simulink model "forGenerate"  (R2015b)
settings: Solver=FixedStepAuto  StartTime=0  StopTime=13  FixedStep=10*(1e-3)  RelTol=1e-3
undefined symbols (not defined in the file or in its folder): qc
libraries: simulink x4
settings Model: Creator=acsl  LastModifiedBy=acsl
settings OptimizationCC: DefaultParameterBehavior=Inlined  UseFloatMulNetSlope=on  InlineInvariantSignals=on  PassReuseOutputArgsAs=Individual arguments  ZeroExternalMemoryAtStartup=off  ZeroInternalMemoryAtStartup=off  NoFixptDivByZeroProtection=on  EfficientFloat2IntCast=on  OptimizeModelRefInitCode=on  LifeSpan=1
settings HardwareCC: ProdBitPerPointer=32  ProdLargestAtomicInteger=Long  ProdLargestAtomicFloat=Double  ProdWordSize=32  ProdHWDeviceType=ARM Compatible->ARM Cortex
settings RTWCC: SystemTargetFile=ert.tlc  TemplateMakefile=ert_default_tmf  Description=Embedded Coder  GenerateReport=on  IncludeHyperlinkInReport=on  LaunchReport=on  GenerateTraceInfo=on  GenerateTraceReport=on  GenerateTraceReportSl=on  GenerateTraceReportSf=on  GenerateTraceReportEml=on  GenerateCodeMetricsReport=on
settings CodeAppCC: ForceParamTrailComments=on  IgnoreCustomStorageClasses=off  SimulinkDataObjDesc=on  CustomSymbolStrGlobalVar=rt$N$M  CustomSymbolStrType=$N$M  CustomSymbolStrFcn=$N$M$F  CustomSymbolStrMacro=$N$M  InsertBlockDesc=on
settings ERTTargetCC: GenerateSampleERTMain=on  IncludeMdlTerminateFcn=off  CombineSignalStateStructs=on  SupportContinuousTime=on  InlinedParameterPlacement=NonHierarchical  ERTCustomFileTemplate=example_file_process.tlc  ERTFilePackagingFormat=CompactWithDataFile

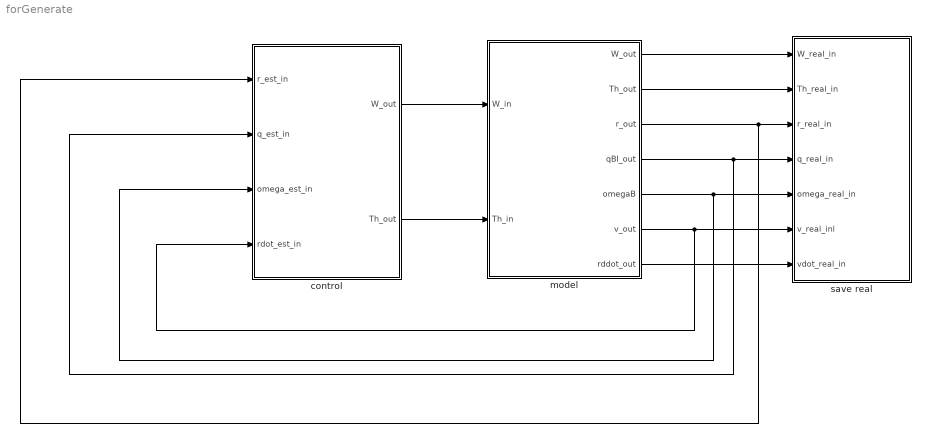
== system forGenerate ==
  control : Subsystem  InitFcn=init
  model : Subsystem
  save real : Subsystem
  wires:
  model/1(W_out) -> save real/1(W_real_in)
  model/2(Th_out) -> save real/2(Th_real_in)
  model/7(rddot_out) -> save real/7(vdot_real_in)
  model/5(omegaB) -> control/3(omega_est_in), save real/5(omega_real_in)
  control/1(W_out) -> model/1(W_in)
  control/2(Th_out) -> model/2(Th_in)
  model/3(r_out) -> control/1(r_est_in), save real/3(r_real_in)
  model/4(qBI_out) -> control/2(q_est_in), save real/4(q_real_in)
  model/6(v_out) -> control/4(rdot_est_in), save real/6(v_real_inl)

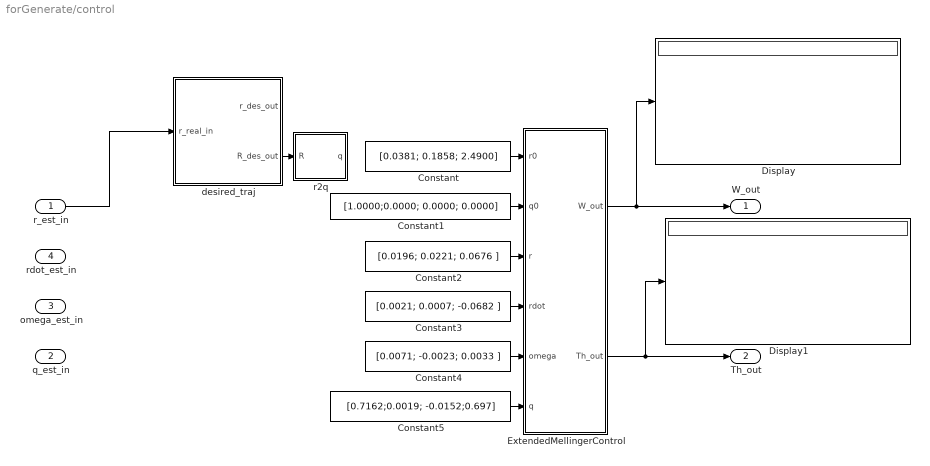
== system forGenerate/control ==
  r_est_in : Inport
  q_est_in : Inport  Port=2
  omega_est_in : Inport  Port=3
  rdot_est_in : Inport  Port=4
  Constant : Constant  Value=[0.0381; 0.1858; 2.4900]  VectorParams1D=off
  Constant1 : Constant  Value=[1.0000;0.0000; 0.0000; 0.0000]  VectorParams1D=off
  Constant2 : Constant  Value=[0.0196; 0.0221; 0.0676 ]  VectorParams1D=off
  Constant3 : Constant  Value=[0.0021; 0.0007; -0.0682 ]  VectorParams1D=off
  Constant4 : Constant  Value=[0.0071; -0.0023; 0.0033 ]
  Constant5 : Constant  Value=[0.7162;0.0019; -0.0152;0.697]  VectorParams1D=off
  Display : Display
  Display1 : Display
  ExtendedMellingerControl : Subsystem
  desired_traj : Subsystem
  r2q : MATLAB Function  TreatAsAtomicUnit=on
  W_out : Outport
  Th_out : Outport  Port=2
  wires:
  r_est_in/1 -> desired_traj/1(r_real_in)
  desired_traj/2(R_des_out) -> r2q/1(R)
  ExtendedMellingerControl/2(Th_out) -> Display1/1, Th_out/1
  Constant/1 -> ExtendedMellingerControl/1(r0)
  Constant1/1 -> ExtendedMellingerControl/2(q0)
  Constant2/1 -> ExtendedMellingerControl/3(r)
  Constant3/1 -> ExtendedMellingerControl/4(rdot)
  Constant4/1 -> ExtendedMellingerControl/5(omega)
  Constant5/1 -> ExtendedMellingerControl/6(q)
  ExtendedMellingerControl/1(W_out) -> Display/1, W_out/1

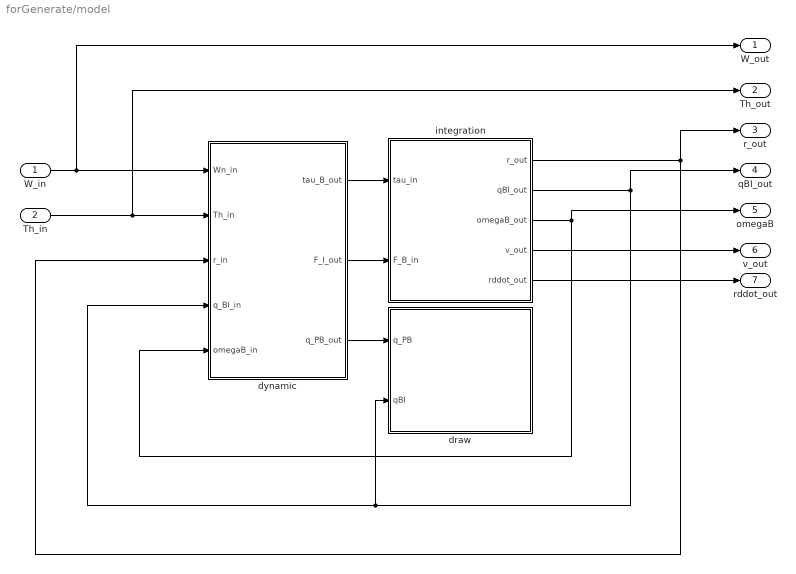
== system forGenerate/model ==
  W_in : Inport
  Th_in : Inport  Port=2
  draw : Subsystem
  dynamic : Subsystem  StopFcn=close all
  integration : Subsystem
  W_out : Outport
  Th_out : Outport  Port=2
  r_out : Outport  Port=3
  qBI_out : Outport  Port=4
  omegaB : Outport  Port=5
  v_out : Outport  Port=6
  rddot_out : Outport  Port=7
  wires:
  integration/1(r_out) -> dynamic/3(r_in), r_out/1
  dynamic/2(F_I_out) -> integration/2(F_B_in)
  integration/2(qBI_out) -> dynamic/4(q_BI_in), draw/2(qBI), qBI_out/1
  W_in/1 -> W_out/1, dynamic/1(Wn_in)
  dynamic/1(tau_B_out) -> integration/1(tau_in)
  integration/3(omegaB_out) -> dynamic/5(omegaB_in), omegaB/1
  Th_in/1 -> dynamic/2(Th_in), Th_out/1
  dynamic/3(q_PB_out) -> draw/1(q_PB)
  integration/4(v_out) -> v_out/1
  integration/5(rddot_out) -> rddot_out/1

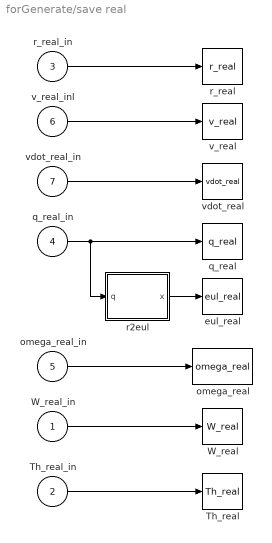
== system forGenerate/save real ==
  W_real_in : Inport
  Th_real_in : Inport  Port=2
  r_real_in : Inport  Port=3
  q_real_in : Inport  Port=4
  omega_real_in : Inport  Port=5
  v_real_inl : Inport  Port=6
  vdot_real_in : Inport  Port=7
  Th_real : ToWorkspace  VariableName=Th_real  SaveFormat=Timeseries  SampleTime=-1
  W_real : ToWorkspace  VariableName=W_real  SaveFormat=Timeseries  SampleTime=-1
  eul_real : ToWorkspace  VariableName=eul_real  SaveFormat=Timeseries  SampleTime=-1
  omega_real : ToWorkspace  VariableName=omega_real  SaveFormat=Timeseries  SampleTime=-1
  q_real : ToWorkspace  VariableName=q_real  SaveFormat=Timeseries  SampleTime=-1
  r2eul : MATLAB Function  TreatAsAtomicUnit=on
  r_real : ToWorkspace  VariableName=r_real  SaveFormat=Timeseries  SampleTime=-1
  v_real : ToWorkspace  VariableName=v_real  SaveFormat=Timeseries  SampleTime=-1
  vdot_real : ToWorkspace  VariableName=vdot_real  SaveFormat=Timeseries  SampleTime=-1
  wires:
  q_real_in/1 -> q_real/1, r2eul/1(q)
  r_real_in/1 -> r_real/1
  v_real_inl/1 -> v_real/1
  vdot_real_in/1 -> vdot_real/1
  r2eul/1(x) -> eul_real/1
  omega_real_in/1 -> omega_real/1
  Th_real_in/1 -> Th_real/1
  W_real_in/1 -> W_real/1

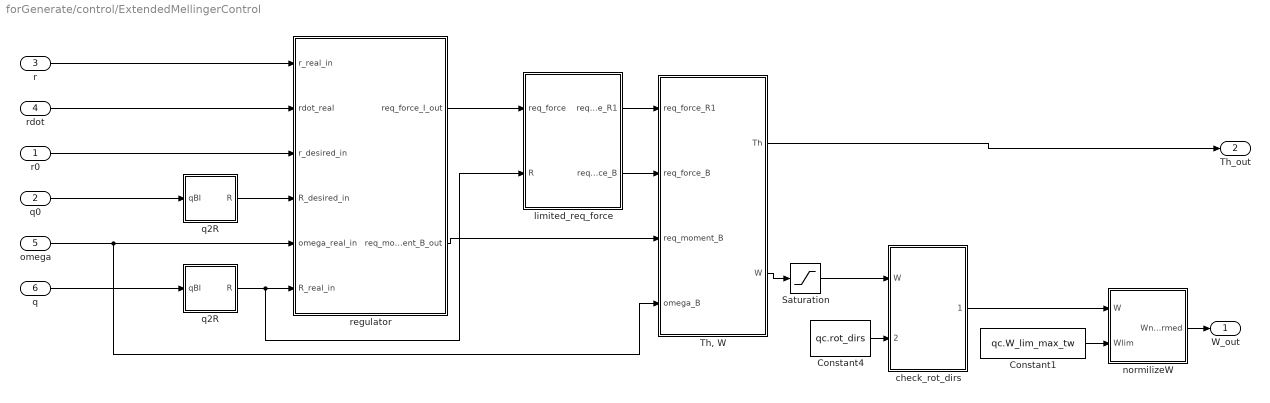
== system forGenerate/control/ExtendedMellingerControl ==
  r0 : Inport
  q0 : Inport  Port=2
  r : Inport  Port=3
  rdot : Inport  Port=4
  omega : Inport  Port=5
  q : Inport  Port=6
  Constant1 : Constant  Value=qc.W_lim_max_tw
  Constant4 : Constant  Value=qc.rot_dirs
  Saturation : Saturate  UpperLimit=qc.W_lim  LowerLimit=-qc.W_lim
  "Th, W" : Subsystem
  check_rot_dirs : MATLAB Function  TreatAsAtomicUnit=on
  limited_req_force : Subsystem
  normilizeW : MATLAB Function  TreatAsAtomicUnit=on
  q2R : MATLAB Function  TreatAsAtomicUnit=on
  "q2R " : MATLAB Function  TreatAsAtomicUnit=on
  regulator : Subsystem
  W_out : Outport
  Th_out : Outport  Port=2
  wires:
  rdot/1 -> regulator/2(rdot_real)
  r0/1 -> regulator/3(r_desired_in)
  r/1 -> regulator/1(r_real_in)
  q0/1 -> "q2R "/1(qBI)
  omega/1 -> regulator/5(omega_real_in), "Th, W"/4(omega_B)
  q/1 -> q2R/1(qBI)
  regulator/2(req_moment_B_out) -> "Th, W"/3(req_moment_B)
  limited_req_force/2(req_force_B) -> "Th, W"/2(req_force_B)
  regulator/1(req_force_I_out) -> limited_req_force/1(req_force)
  q2R/1(R) -> limited_req_force/2(R), regulator/6(R_real_in)
  limited_req_force/1(req_force_R1) -> "Th, W"/1(req_force_R1)
  "Th, W"/1(Th) -> Th_out/1
  "Th, W"/2(W) -> Saturation/1
  Constant1/1 -> normilizeW/2(Wlim)
  normilizeW/1(Wnormed) -> W_out/1
  Constant4/1 -> check_rot_dirs/2(rot_dirs)
  Saturation/1 -> check_rot_dirs/1(W)
  check_rot_dirs/1(W_directed) -> normilizeW/1(W)
  "q2R "/1(R) -> regulator/4(R_desired_in)

== system forGenerate/control/desired_traj ==
  r_real_in : Inport
  To Workspace1 : ToWorkspace  VariableName=time  SaveFormat=Timeseries  SampleTime=-1
  To Workspace2 : ToWorkspace  VariableName=r_des  SaveFormat=Timeseries  SampleTime=-1
  To Workspace6 : ToWorkspace  VariableName=eul_des  SaveFormat=Timeseries  SampleTime=-1
  time : simulink/Sources/Ramp  slope=1  start=0  X0=0
  traj : MATLAB Function  TreatAsAtomicUnit=on
  r_des_out : Outport
  R_des_out : Outport  Port=2
  wires:
  traj/2(R_des) -> R_des_out/1
  time/1 -> To Workspace1/1, traj/1(t)
  traj/3(eul_des) -> To Workspace6/1
  r_real_in/1 -> traj/2(rr)
  traj/1(r_des) -> To Workspace2/1, r_des_out/1

== system forGenerate/model/draw ==
  q_PB : Inport
  qBI : Inport  Port=2
  Constant : Constant  Value=qc.rays
  Constant1 : Constant  Value=qc.l
  Constant2 : Constant  Value=qc.draw_mode
  Rate Transition : RateTransition
  Rate Transition1 : RateTransition
  draw : MATLAB Function  TreatAsAtomicUnit=on  SystemSampleTime=qc.draw_tick
  wires:
  Constant1/1 -> draw/4(l)
  q_PB/1 -> Rate Transition1/1
  Rate Transition1/1 -> draw/2(q_PB)
  Constant/1 -> draw/3(rays)
  Rate Transition/1 -> draw/1(q_BI)
  qBI/1 -> Rate Transition/1
  Constant2/1 -> draw/5(draw_mode)

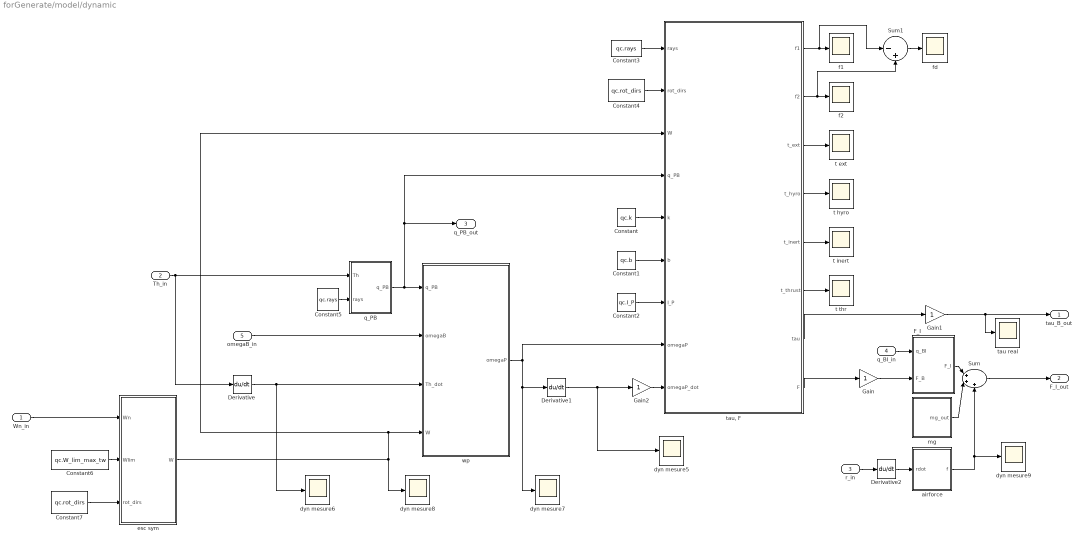
== system forGenerate/model/dynamic ==
  Wn_in : Inport
  Th_in : Inport  Port=2
  r_in : Inport  Port=3
  q_BI_in : Inport  Port=4
  omegaB_in : Inport  Port=5
  Constant : Constant  Value=qc.k
  Constant1 : Constant  Value=qc.b
  Constant2 : Constant  Value=qc.I_P
  Constant3 : Constant  Value=qc.rays
  Constant4 : Constant  Value=qc.rot_dirs
  Constant5 : Constant  Value=qc.rays
  Constant6 : Constant  Value=qc.W_lim_max_tw
  Constant7 : Constant  Value=qc.rot_dirs
  Derivative : Derivative
  Derivative1 : Derivative
  Derivative2 : Derivative
  F_I : MATLAB Function  TreatAsAtomicUnit=on
  Gain : Gain
  Gain1 : Gain
  Gain2 : Gain
  Sum : Sum  Inputs=|+++
  Sum1 : Sum  Inputs=|-+
  airforce : Subsystem
  dyn mesure{5..9} (5 alike) : Scope
  esc sym : MATLAB Function  TreatAsAtomicUnit=on
  f1 : Scope
  f2 : Scope
  fd : Scope
  mg : Subsystem
  q_PB : MATLAB Function  TreatAsAtomicUnit=on
  t ext : Scope
  t hyro : Scope
  t inert : Scope
  t thr : Scope
  tau real : Scope
  "tau, F" : MATLAB Function  TreatAsAtomicUnit=on
  wp : MATLAB Function  TreatAsAtomicUnit=on
  tau_B_out : Outport
  F_I_out : Outport  Port=2
  q_PB_out : Outport  Port=3
  wires:
  Th_in/1 -> Derivative/1, q_PB/1(Th)
  q_PB/1(q_PB) -> "tau, F"/4(q_PB), q_PB_out/1, wp/1(q_PB)
  omegaB_in/1 -> wp/2(omegaB)
  wp/1(omegaP) -> dyn mesure7/1, Derivative1/1, "tau, F"/8(omegaP)
  Constant/1 -> "tau, F"/5(k)
  Constant1/1 -> "tau, F"/6(b)
  Constant2/1 -> "tau, F"/7(I_P)
  "tau, F"/8(F) -> Gain/1
  Constant3/1 -> "tau, F"/1(rays)
  Constant4/1 -> "tau, F"/2(rot_dirs)
  Constant5/1 -> q_PB/2(rays)
  q_BI_in/1 -> F_I/1(q_BI)
  Gain/1 -> F_I/2(F_B)
  F_I/1(F_I) -> Sum/1
  mg/1(mg_out) -> Sum/2
  Sum/1 -> F_I_out/1
  r_in/1 -> Derivative2/1
  airforce/1(f) -> dyn mesure9/1, Sum/3
  "tau, F"/7(tau) -> Gain1/1
  Derivative2/1 -> airforce/1(rdot)
  "tau, F"/3(t_ext) -> t ext/1
  "tau, F"/4(t_hyro) -> t hyro/1
  "tau, F"/5(t_inert) -> t inert/1
  "tau, F"/6(t_thrust) -> t thr/1
  Gain2/1 -> "tau, F"/9(omegaP_dot)
  Derivative/1 -> wp/3(Th_dot), dyn mesure6/1
  esc sym/1(W) -> wp/4(W), "tau, F"/3(W), dyn mesure8/1
  Derivative1/1 -> dyn mesure5/1, Gain2/1
  Gain1/1 -> tau_B_out/1, tau real/1
  "tau, F"/1(f1) -> Sum1/1, f1/1
  "tau, F"/2(f2) -> Sum1/2, f2/1
  Sum1/1 -> fd/1
  Constant6/1 -> esc sym/2(Wlim)
  Constant7/1 -> esc sym/3(rot_dirs)
  Wn_in/1 -> esc sym/1(Wn)

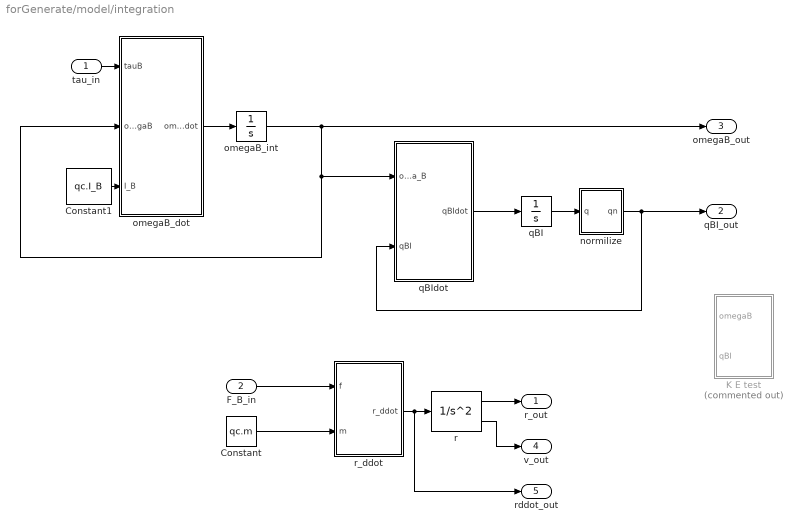
== system forGenerate/model/integration ==
  tau_in : Inport
  F_B_in : Inport  Port=2
  Constant : Constant  Value=qc.m
  Constant1 : Constant  Value=qc.I_B
  K E test : Subsystem  Commented=on
  normilize : MATLAB Function  TreatAsAtomicUnit=on
  omegaB_dot : MATLAB Function  TreatAsAtomicUnit=on
  omegaB_int : Integrator  InitialCondition=qc.omegaB0
  qBI : Integrator  InitialCondition=qc.qBI0
  qBIdot : MATLAB Function  TreatAsAtomicUnit=on
  r : SecondOrderIntegrator  ICX=qc.r0  ICDXDT=qc.v0
  r_ddot : MATLAB Function  TreatAsAtomicUnit=on
  r_out : Outport
  qBI_out : Outport  Port=2
  omegaB_out : Outport  Port=3
  v_out : Outport  Port=4
  rddot_out : Outport  Port=5
  wires:
  r/1 -> r_out/1
  r_ddot/1(r_ddot) -> rddot_out/1, r/1
  Constant/1 -> r_ddot/2(m)
  omegaB_int/1 -> omegaB_out/1, qBIdot/1(omega_B), omegaB_dot/2(omegaB)
  Constant1/1 -> omegaB_dot/3(I_B)
  tau_in/1 -> omegaB_dot/1(tauB)
  qBIdot/1(qBIdot) -> qBI/1
  qBI/1 -> normilize/1(q)
  normilize/1(qn) -> qBI_out/1, qBIdot/2(qBI)
  F_B_in/1 -> r_ddot/1(f)
  omegaB_dot/1(omegaB_dot) -> omegaB_int/1
  r/2 -> v_out/1

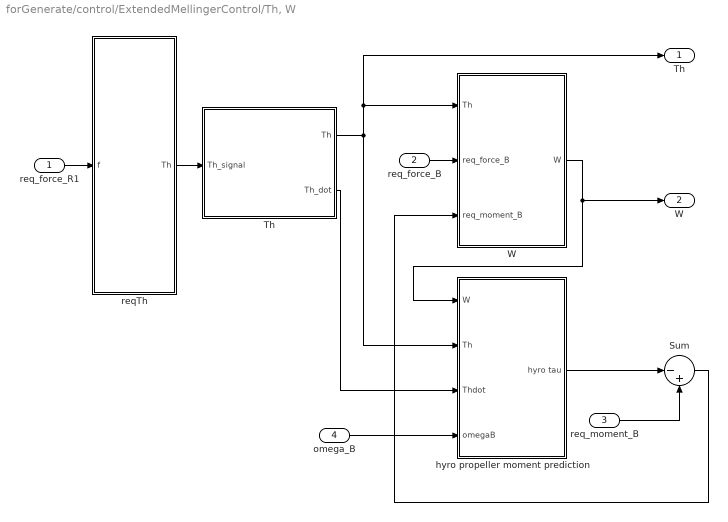
== system forGenerate/control/ExtendedMellingerControl/Th, W ==
  req_force_R1 : Inport
  req_force_B : Inport  Port=2
  req_moment_B : Inport  Port=3
  omega_B : Inport  Port=4
  Sum : Sum  Inputs=|-+
  "Th " : Subsystem
  "W " : Subsystem
  hyro propeller moment prediction : Subsystem
  reqTh : MATLAB Function  TreatAsAtomicUnit=on
  Th : Outport
  W : Outport  Port=2
  wires:
  req_force_B/1 -> "W "/2(req_force_B)
  req_force_R1/1 -> reqTh/1(f)
  "Th "/1(Th) -> hyro propeller moment prediction/2(Th), Th/1, "W "/1(Th)
  reqTh/1(Th) -> "Th "/1(Th_signal)
  "W "/1(W) -> hyro propeller moment prediction/1(W), W/1
  omega_B/1 -> hyro propeller moment prediction/4(omegaB)
  "Th "/2(Th_dot) -> hyro propeller moment prediction/3(Thdot)
  req_moment_B/1 -> Sum/2
  hyro propeller moment prediction/1(hyro tau) -> Sum/1
  Sum/1 -> "W "/3(req_moment_B)

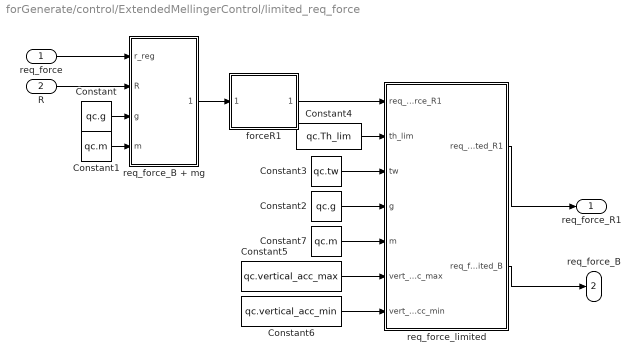
== system forGenerate/control/ExtendedMellingerControl/limited_req_force ==
  req_force : Inport
  R : Inport  Port=2
  Constant : Constant  Value=qc.g
  Constant1 : Constant  Value=qc.m
  Constant2 : Constant  Value=qc.g
  Constant3 : Constant  Value=qc.tw
  Constant4 : Constant  Value=qc.Th_lim
  Constant5 : Constant  Value=qc.vertical_acc_max
  Constant6 : Constant  Value=qc.vertical_acc_min
  Constant7 : Constant  Value=qc.m
  forceR1 : MATLAB Function  TreatAsAtomicUnit=on
  req_force_B + mg : MATLAB Function  TreatAsAtomicUnit=on
  req_force_limited : MATLAB Function  TreatAsAtomicUnit=on
  req_force_R1 : Outport
  req_force_B : Outport  Port=2
  wires:
  R/1 -> req_force_B + mg/2(R)
  Constant3/1 -> req_force_limited/3(tw)
  forceR1/1(force_R1) -> req_force_limited/1(req_force_R1)
  Constant1/1 -> req_force_B + mg/4(m)
  Constant7/1 -> req_force_limited/5(m)
  Constant/1 -> req_force_B + mg/3(g)
  Constant4/1 -> req_force_limited/2(th_lim)
  req_force_limited/2(req_force_limited_B) -> req_force_B/1
  req_force_limited/1(req_force_limited_R1) -> req_force_R1/1
  Constant2/1 -> req_force_limited/4(g)
  req_force/1 -> req_force_B + mg/1(r_reg)
  req_force_B + mg/1(r_reg_translated) -> forceR1/1(req_force_B)
  Constant5/1 -> req_force_limited/6(vert_acc_max)
  Constant6/1 -> req_force_limited/7(vert_acc_min)

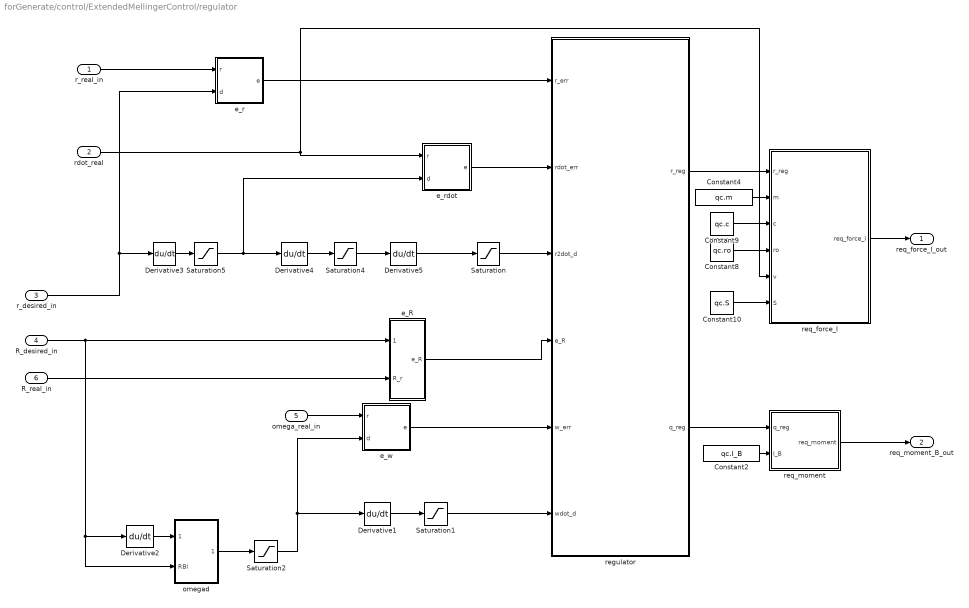
== system forGenerate/control/ExtendedMellingerControl/regulator ==
  r_real_in : Inport
  rdot_real : Inport  Port=2
  r_desired_in : Inport  Port=3
  R_desired_in : Inport  Port=4
  omega_real_in : Inport  Port=5
  R_real_in : Inport  Port=6
  Constant10 : Constant  Value=qc.S
  Constant2 : Constant  Value=qc.I_B
  Constant4 : Constant  Value=qc.m
  Constant8 : Constant  Value=qc.ro
  Constant9 : Constant  Value=qc.c
  Derivative{1..5} (5 alike) : Derivative
  Saturation : Saturate  UpperLimit=qc.r2dot_des_lim  LowerLimit=-qc.r2dot_des_lim
  Saturation1 : Saturate  UpperLimit=qc.w_des_lim/2  LowerLimit=-qc.w_des_lim/2
  Saturation2 : Saturate  UpperLimit=qc.w_des_lim  LowerLimit=-qc.w_des_lim
  Saturation4 : Saturate  UpperLimit=qc.r2dot_des_lim  LowerLimit=-qc.r2dot_des_lim
  Saturation5 : Saturate  UpperLimit=qc.rdot_des_lim  LowerLimit=-qc.rdot_des_lim
  e_R : MATLAB Function  TreatAsAtomicUnit=on
  e_r : MATLAB Function  TreatAsAtomicUnit=on
  e_rdot : MATLAB Function  TreatAsAtomicUnit=on
  e_w : MATLAB Function  TreatAsAtomicUnit=on
  omegad : MATLAB Function  TreatAsAtomicUnit=on
  regulator : MATLAB Function  TreatAsAtomicUnit=on
  req_force_I : MATLAB Function  TreatAsAtomicUnit=on
  req_moment : MATLAB Function  TreatAsAtomicUnit=on
  req_force_I_out : Outport
  req_moment_B_out : Outport  Port=2
  wires:
  Saturation1/1 -> regulator/6(wdot_d)
  Derivative1/1 -> Saturation1/1
  Saturation/1 -> regulator/3(r2dot_d)
  R_real_in/1 -> e_R/2(R_r)
  Saturation5/1 -> Derivative4/1, e_rdot/2(d)
  Saturation4/1 -> Derivative5/1
  Saturation2/1 -> e_w/2(d), Derivative1/1
  r_desired_in/1 -> e_r/2(d), Derivative3/1
  r_real_in/1 -> e_r/1(r)
  omega_real_in/1 -> e_w/1(r)
  e_w/1(e) -> regulator/5(w_err)
  Derivative5/1 -> Saturation/1
  rdot_real/1 -> req_force_I/5(v), e_rdot/1(r)
  e_rdot/1(e) -> regulator/2(rdot_err)
  e_r/1(e) -> regulator/1(r_err)
  Derivative4/1 -> Saturation4/1
  e_R/1(e_R) -> regulator/4(e_R)
  Derivative3/1 -> Saturation5/1
  omegad/1(omega) -> Saturation2/1
  R_desired_in/1 -> e_R/1(R_d), Derivative2/1, omegad/2(RBI)
  Derivative2/1 -> omegad/1(RBIdot)
  regulator/2(q_reg) -> req_moment/1(q_reg)
  req_moment/1(req_moment) -> req_moment_B_out/1
  Constant2/1 -> req_moment/2(I_B)
  regulator/1(r_reg) -> req_force_I/1(r_reg)
  req_force_I/1(req_force_I) -> req_force_I_out/1
  Constant4/1 -> req_force_I/2(m)
  Constant9/1 -> req_force_I/3(c)
  Constant10/1 -> req_force_I/6(S)
  Constant8/1 -> req_force_I/4(ro)

== system forGenerate/model/dynamic/airforce ==
  rdot : Inport
  Constant10 : Constant  Value=qc.S
  Constant8 : Constant  Value=qc.ro
  Constant9 : Constant  Value=qc.c
  air force I : MATLAB Function  TreatAsAtomicUnit=on
  f : Outport
  wires:
  air force I/1(f) -> f/1
  Constant9/1 -> air force I/3(c)
  Constant10/1 -> air force I/4(S)
  Constant8/1 -> air force I/2(ro)
  rdot/1 -> air force I/1(r_dot)

== system forGenerate/model/dynamic/mg ==
  Constant6 : Constant  Value=qc.m
  Constant7 : Constant  Value=qc.g
  mg : MATLAB Function  TreatAsAtomicUnit=on
  mg_out : Outport
  wires:
  Constant7/1 -> mg/2(g)
  Constant6/1 -> mg/1(m)
  mg/1(mg) -> mg_out/1

== system forGenerate/model/integration/K E test ==
  omegaB : Inport
  qBI : Inport  Port=2
  Constant2 : Constant  Value=qc.I_B
  "K, E" : MATLAB Function  TreatAsAtomicUnit=on
  rgb : Scope
  rgb1 : Scope
  wires:
  omegaB/1 -> "K, E"/2(omega_B)
  qBI/1 -> "K, E"/3(qBI)
  "K, E"/1(K) -> rgb/1
  "K, E"/2(E) -> rgb1/1
  Constant2/1 -> "K, E"/1(I_B)

== system forGenerate/control/ExtendedMellingerControl/Th, W/Th  ==
  Th_signal : Inport
  Demux : Demux
  Derivative : Derivative
  Mux : Mux
  Transfer Fcn{,1..3} (4 alike) : TransferFcn  Numerator=qc.Th_transfer_top  Denominator=qc.Th_transfer_bot
  Th : Outport
  Th_dot : Outport  Port=2
  wires:
  Demux/1 -> Transfer Fcn/1
  Transfer Fcn/1 -> Mux/1
  Demux/2 -> Transfer Fcn1/1
  Demux/3 -> Transfer Fcn2/1
  Demux/4 -> Transfer Fcn3/1
  Transfer Fcn1/1 -> Mux/2
  Transfer Fcn2/1 -> Mux/3
  Transfer Fcn3/1 -> Mux/4
  Mux/1 -> Derivative/1, Th/1
  Th_signal/1 -> Demux/1
  Derivative/1 -> Th_dot/1

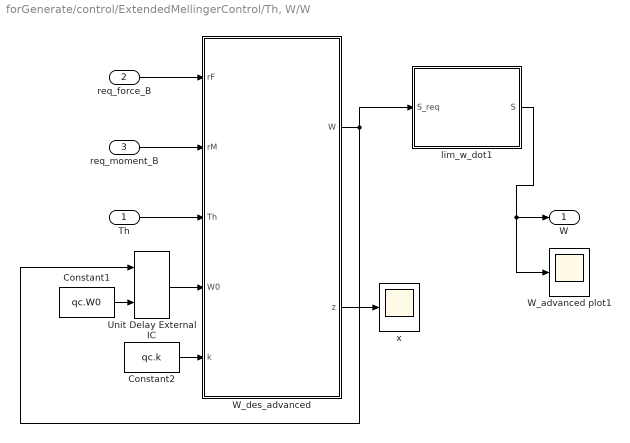
== system forGenerate/control/ExtendedMellingerControl/Th, W/W  ==
  Th : Inport
  req_force_B : Inport  Port=2
  req_moment_B : Inport  Port=3
  Constant1 : Constant  Value=qc.W0
  Constant2 : Constant  Value=qc.k
  Unit Delay External IC : simulink/Additional Math & Discrete/Additional Discrete/Unit Delay External IC  tsamp=-1
  W_advanced plot1 : Scope
  W_des_advanced : MATLAB Function  TreatAsAtomicUnit=on
  lim_w_dot1 : Subsystem
  x : Scope
  W : Outport
  wires:
  Th/1 -> W_des_advanced/3(Th)
  W_des_advanced/1(W) -> lim_w_dot1/1(S_req), Unit Delay External IC/1
  Constant1/1 -> Unit Delay External IC/2
  Unit Delay External IC/1 -> W_des_advanced/4(W0)
  Constant2/1 -> W_des_advanced/5(k)
  lim_w_dot1/1(S) -> W_advanced plot1/1, W/1
  req_force_B/1 -> W_des_advanced/1(rF)
  req_moment_B/1 -> W_des_advanced/2(rM)
  W_des_advanced/2(z) -> x/1

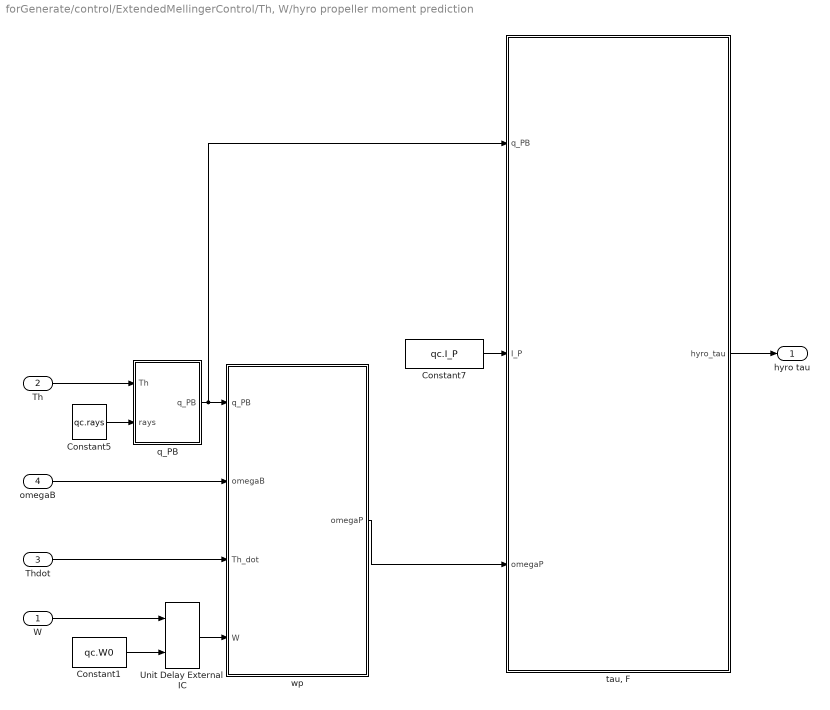
== system forGenerate/control/ExtendedMellingerControl/Th, W/hyro propeller moment prediction ==
  W : Inport
  Th : Inport  Port=2
  Thdot : Inport  Port=3
  omegaB : Inport  Port=4
  Constant1 : Constant  Value=qc.W0
  Constant5 : Constant  Value=qc.rays
  Constant7 : Constant  Value=qc.I_P
  Unit Delay External IC : simulink/Additional Math & Discrete/Additional Discrete/Unit Delay External IC  tsamp=-1
  q_PB : MATLAB Function  TreatAsAtomicUnit=on
  "tau, F" : MATLAB Function  TreatAsAtomicUnit=on
  wp : MATLAB Function  TreatAsAtomicUnit=on
  hyro tau : Outport
  wires:
  q_PB/1(q_PB) -> wp/1(q_PB), "tau, F"/1(q_PB)
  W/1 -> Unit Delay External IC/1
  "tau, F"/1(hyro_tau) -> hyro tau/1
  Th/1 -> q_PB/1(Th)
  Constant1/1 -> Unit Delay External IC/2
  Thdot/1 -> wp/3(Th_dot)
  wp/1(omegaP) -> "tau, F"/3(omegaP)
  Constant5/1 -> q_PB/2(rays)
  Unit Delay External IC/1 -> wp/4(W)
  omegaB/1 -> wp/2(omegaB)
  Constant7/1 -> "tau, F"/2(I_P)

== system forGenerate/control/ExtendedMellingerControl/Th, W/W /lim_w_dot1 ==
  S_req : Inport
  Constant2 : Constant  Value=qc.w_dot_lim
  Constant3 : Constant  Value=qc.time_step
  Derivative : Derivative
  Unit Delay External IC : simulink/Additional Math & Discrete/Additional Discrete/Unit Delay External IC  tsamp=-1
  W to w : MATLAB Function  TreatAsAtomicUnit=on
  limit w dot : MATLAB Function  TreatAsAtomicUnit=on
  u plot1 : Scope
  u plot2 : Scope
  w to W : MATLAB Function  TreatAsAtomicUnit=on
  S : Outport
  wires:
  Derivative/1 -> u plot2/1
  limit w dot/1(lim_S) -> w to W/1(w), Derivative/1, Unit Delay External IC/1
  w to W/1(W) -> S/1
  W to w/1(w) -> limit w dot/2(S_req), Unit Delay External IC/2, u plot1/1
  Constant3/1 -> limit w dot/4(dt)
  S_req/1 -> W to w/1(W)
  Unit Delay External IC/1 -> limit w dot/1(S0)
  Constant2/1 -> limit w dot/3(S_dot_lim)

== matlab function forGenerate/model/dynamic/wp ==
  data: q_PB input; omegaP output; omegaB input; Th_dot input; W input
function omegaP  = fcn(q_PB, omegaB, Th_dot, W)

omegaP = zeros(4*3,1);
for i = 1:4
    q_pb = q_PB(:, i);
    q_bp = quatDual(q_pb);
    w = sign(W(i))*sqrt(abs(W(i)));
    omegaP(3*i-2:3*i, 1) = quatRotate(q_bp, omegaB) + [Th_dot(i); 0; w];
end

== matlab function forGenerate/model/integration/normilize ==
  data: q input; qn output
function qn  = fcn(q)
qn = q / norm(q);

== matlab function forGenerate/model/dynamic/tau, F ==
  data: f1 output; f2 output; t_ext output; t_hyro output; t_inert output; t_thrust output; rays input; rot_dirs input; W input; q_PB input; k input; b input; I_P input; omegaP input; omegaP_dot input; tau output; F output
function [f1, f2, t_ext,t_hyro, t_inert, t_thrust, tau, F]= fcn(rays, rot_dirs, W, q_PB, k, b, I_P, omegaP, omegaP_dot)

tau = [0;0;0];
F = [0;0;0];

t_ext = [0;0;0];
t_hyro = [0;0;0];
t_inert = [0;0;0];
t_thrust = [0;0;0];

f1 = 0;
f2 = 0;
for i = 1:4
    ray = rays(3*i-2:3*i);
    dir = rot_dirs(i);  
    omega_p = omegaP(3*i-2:3*i);
    omega_pz = omega_p(3);
    omega_p_dot = omegaP_dot(3*i-2:3*i);
    q_pb = q_PB(:, i);

    fp = dir*[0;0;k*W(i)];
    fb = quatRotate(q_pb,fp);
    
    if i == 1 || i ==3
        f1 = f1 + fb(3);
    else
        f2 = f2 + fb(3);
    end
    
    tau_p_ext = [0;0;-b*abs(omega_pz)*omega_pz];
    tau_p = 1*I_P*omega_p_dot + 1*cross(omega_p, I_P*omega_p) - tau_p_ext; %%%%%%% 1 !!!!!!!!!!!!
    tau_b = cross(ray, fb) - quatRotate(q_pb, tau_p);
    
    tau = tau + tau_b;  
    F = F + fb;
    
    t_ext = t_ext + quatRotate(q_pb,tau_p_ext);
    t_hyro = t_hyro + quatRotate(q_pb, cross(omega_p, I_P*omega_p));
    t_inert = t_inert + quatRotate(q_pb,I_P*omega_p_dot);
    t_thrust = t_thrust + cross(ray, fb);
    
end

== matlab function forGenerate/control/ExtendedMellingerControl/regulator/e_R ==
  data: R_d input; R_r input; e_R output size=3
function e_R = e_r(R_d, R_r)
Me_R = R_r'*R_d - R_d'*R_r;
e_R = 0.5*[-Me_R(2,3); Me_R(1,3); -Me_R(1,2)];
end

== matlab function forGenerate/model/dynamic/mg/mg ==
  data: m input; mg output; g input
function mg  = fcn(m, g)
mg = m*g;

== matlab function forGenerate/model/integration/r_ddot ==
  data: r_ddot output; f input; m input
function r_ddot  = fcn(f, m)

r_ddot = f/m;

== matlab function forGenerate/save real/r2eul ==
  data: q input; x output
function x = fnc(q)
eul = quat2eul(q');
x = eul';
end

== matlab function forGenerate/model/integration/omegaB_dot ==
  data: tauB input; omegaB_dot output; omegaB input; I_B input
function omegaB_dot  = fcn(tauB, omegaB, I_B)
omegaB_dot = I_B^(-1) * (tauB - 1*cross(omegaB, I_B * omegaB));

== matlab function forGenerate/model/dynamic/F_I ==
  data: q_BI input; F_I output; F_B input
function F_I  = fcn(q_BI, F_B)
F_I = quatRotate(q_BI, F_B);

== matlab function forGenerate/model/integration/qBIdot ==
  data: omega_B input; qBIdot output; qBI input
function qBIdot  = fcn(omega_B, qBI)
qw = [0;omega_B];
qBIdot = 0.5*quatMultiply(qBI, qw);

== matlab function forGenerate/control/ExtendedMellingerControl/regulator/e_r ==
  data: r input; d input; e output size=3
function e = e_r(r, d)
e = d - r;

== matlab function forGenerate/model/draw/draw ==
  data: q_BI input; q_PB input; rays input; l input; draw_mode input
function drawFly(q_BI, q_PB, rays, l, draw_mode)
drawFly(q_BI, q_PB, rays, l, draw_mode)
end

== matlab function forGenerate/model/integration/K E test/K, E ==
  data: I_B input; omega_B input; qBI input; K output; E output
function [K, E] = fcn(I_B, omega_B, qBI)
K_B = I_B*omega_B;
K = quatRotate(qBI, K_B);
E = omega_B'*I_B*omega_B / 2;

== matlab function forGenerate/control/ExtendedMellingerControl/regulator/e_rdot ==
  data: r input; d input; e output size=3
function e = e_r(r, d)
e = d - r;

== matlab function forGenerate/control/ExtendedMellingerControl/regulator/e_w ==
  data: r input; d input; e output size=3
function e = e_r(r, d)
e = d - r;
end

== matlab function forGenerate/control/ExtendedMellingerControl/regulator/regulator ==
  data: r_err input; rdot_err input; r_reg output; r2dot_d input; e_R input; w_err input; wdot_d input; q_reg output
function [r_reg, q_reg]= x_e(r_err, rdot_err, r2dot_d, e_R, w_err, wdot_d)
   
K1 = [1,0,0;
      0,1,0;
      0,0,1]*120;

K0 =   [1,0,0;
       0,1,0;
       0,0,1]*90;
   
r_reg =  r2dot_d + K1*(rdot_err)+ K0*(r_err);

C1 =   [1,0,0;
        0,1,0;
        0,0,1]*40;

C0 =   [1,0,0;
        0,1,0;
        0,0,1]*40;
          
q_reg = wdot_d + C1*(w_err) + C0*(e_R);
end

== matlab function forGenerate/control/ExtendedMellingerControl/regulator/omegad ==
  data: omega output; RBIdot input; RBI input
function omega  = fcn(RBIdot, RBI)

R = RBI'*RBIdot;
omega = [-R(2,3); R(1,3); -R(1,2)];

== matlab function forGenerate/control/ExtendedMellingerControl/q2R ==
  data: qBI input; R output
function R = q2R(qBI)
R = quat2matrix(qBI);
end

== matlab function forGenerate/control/ExtendedMellingerControl/normilizeW ==
  data: W input; Wnormed output; Wlim input
function Wnormed = fcn(W, Wlim)
Wnormed = zeros(4,1);
for i=1:4
    Wnormed(i) = abs(W(i))/ Wlim;
end
end

== matlab function forGenerate/model/dynamic/esc sym ==
  data: Wn input; W output; Wlim input; rot_dirs input
function W = fcn(Wn, Wlim, rot_dirs)
W = zeros(4,1);
for i=1:4
    W(i) = Wlim*Wn(i)*rot_dirs(i);
end
end

== matlab function forGenerate/control/ExtendedMellingerControl/Th, W/hyro propeller moment prediction/q_PB ==
  data: Th input; q_PB output; rays input
function q_PB = fcn(Th, rays)
q_PB = quatPB(Th, rays);
end

== matlab function forGenerate/control/ExtendedMellingerControl/Th, W/hyro propeller moment prediction/tau, F ==
  data: q_PB input; I_P input; omegaP input; hyro_tau output
function hyro_tau = fcn(q_PB, I_P, omegaP)
hyro_tau = [0;0;0];
for i = 1:4
    omega_p = omegaP(3*i-2:3*i);
    q_pb = q_PB(:, i);
    hyro_tau_P = cross(omega_p, I_P*omega_p);
    hyro_tau = hyro_tau - quatRotate(q_pb, hyro_tau_P);
end

== matlab function forGenerate/control/ExtendedMellingerControl/check_rot_dirs ==
  data: W input; rot_dirs input; W_directed output
function W_directed = translate(W, rot_dirs)
for i = 1:4
    rd = rot_dirs(i);
    if W(i)*rd < 0
        W(i) = 0;
    end
end
W_directed = W;
end

== matlab function forGenerate/control/r2q ==
  data: R input; q output
function q = fcn(R)
q = matrix2quat(R);
end

== matlab function forGenerate/control/desired_traj/traj ==
  data: r_des output; R_des output; t input; eul_des output; rr input
function [r_des, R_des, eul_des] = curve(t, rr)
[ r_des, R_des, eul_des ] = current_traj( t, rr);
end

== matlab function forGenerate/model/dynamic/q_PB ==
  data: Th input; q_PB output; rays input
function q_PB = fcn(Th, rays)
q_PB = quatPB(Th, rays);
end

== matlab function forGenerate/model/dynamic/airforce/air force I ==
  data: r_dot input; f output; ro input; c input; S input
function f = fcn(r_dot, ro, c, S)
f = -ro*c*S*norm(r_dot)*r_dot;

== matlab function forGenerate/control/ExtendedMellingerControl/Th, W/W /W_des_advanced ==
  data: rF input; rM input; Th input; W0 input; k input; W output; z output
function [W, z]= fnc(rF, rM, Th, W0, k)
u = [rF(3); rM(1); rM(2); rM(3)];

Jt = Jt_fcn_advanced(Th(1),Th(2),Th(3),Th(4),W0(1),W0(2),W0(3),W0(4));
f = ft_fcn_advanced(Th(1),Th(2),Th(3),Th(4),W0(1),W0(2),W0(3),W0(4));

u1eq = [k*cos(Th(1)), -k*cos(Th(2)), k*cos(Th(1)), -k*cos(Th(2))];
A = [u1eq; Jt];
Apinv = pinv(A);
B = [zeros(1,4); f];


W = Apinv*(u+B*W0);

q = sqrt(2)/2;
ef1 = [q*sin(Th(1));-q*sin(Th(1));cos(Th(1))];
ef2 = [-q*sin(Th(2));-q*sin(Th(2));-cos(Th(2))];
x = dot(ef1, rM)/3e-6;
y = W(1)+W(3);
z = [x;y];
end

== matlab function forGenerate/control/ExtendedMellingerControl/q2R  ==
  data: qBI input; R output
function R = q2R(qBI)
R = quat2matrix(qBI);
end

== matlab function forGenerate/control/ExtendedMellingerControl/Th, W/W /lim_w_dot1/W to w ==
  data: W input; w output
function w = fnc(W)
w = [0;0;0;0];
for i =1:4
    w(i) = sign(W(i))*sqrt(abs(W(i)));
end
end

== matlab function forGenerate/control/ExtendedMellingerControl/limited_req_force/req_force_B + mg ==
  data: r_reg input; R input; g input; m input; r_reg_translated output
function r_reg_translated = translate(r_reg, R, g, m)
r_reg_translated = R'*(r_reg - m*g);
end

== matlab function forGenerate/control/ExtendedMellingerControl/Th, W/W /lim_w_dot1/limit w dot ==
  data: S0 input; S_req input; lim_S output; S_dot_lim input; dt input
function lim_S = fnc(S0, S_req, S_dot_lim, dt)
S_dot = (S_req-S0)/dt;
for i =1:4
    S_dot(i,1) = set_between(S_dot(i), S_dot_lim, -S_dot_lim);
end
lim_S = S0 +S_dot*dt;
end

== matlab function forGenerate/control/ExtendedMellingerControl/Th, W/W /lim_w_dot1/w to W ==
  data: W output; w input
function W = fnc(w)
W = [0;0;0;0];
for i =1:4
    W(i) = w(i)*abs(w(i));
end
end

== matlab function forGenerate/control/ExtendedMellingerControl/regulator/req_moment ==
  data: q_reg input; req_moment output; I_B input
function req_moment = translate(q_reg, I_B)
req_moment = I_B*q_reg;
end

== matlab function forGenerate/control/ExtendedMellingerControl/limited_req_force/forceR1 ==
  data: req_force_B input; force_R1 output
function force_R1= fcn(req_force_B)

%%
qR1B = quatR1B;
qBR1 = quatDual(qR1B);
force_R1 = quatRotate(qBR1, req_force_B);
end

== matlab function forGenerate/control/ExtendedMellingerControl/limited_req_force/req_force_limited ==
  data: req_force_R1 input; th_lim input; tw input; g input; req_force_limited_R1 output; m input; req_force_limited_B output; vert_acc_max input; vert_acc_min input
function [req_force_limited_R1, req_force_limited_B]= limit(req_force_R1, th_lim, tw, g, m, vert_acc_max, vert_acc_min)
%%
g_abs = abs(g(3));
lim_save_coeff = 0.85;
%%
v_force_max = m*(vert_acc_max + g_abs);
v_force_min = m*(vert_acc_min + g_abs);
force_lim = m*g_abs*tw*lim_save_coeff;
[h_force_lim, req_force_limited_R1] = lim_req_force(req_force_R1, th_lim, force_lim, v_force_max,  v_force_min);
qR1B = quatR1B();
req_force_limited_B = quatRotate(qR1B, req_force_limited_R1);
end

== matlab function forGenerate/control/ExtendedMellingerControl/Th, W/reqTh ==
  data: f input; Th output
function Th = fcn(f)
tgTh24 = 2*f(1)/f(3);
tgTh13 = 2*f(2)/f(3);
Th13 = atan(tgTh13);
Th24 = atan(tgTh24);
Th = [-Th13; Th24; Th13; -Th24];
end

== matlab function forGenerate/control/ExtendedMellingerControl/regulator/req_force_I ==
  data: r_reg input; req_force_I output; m input; c input; ro input; v input; S input
function req_force_I = translate(r_reg, m, c, ro, v, S)
req_force_I = m*r_reg + 0.5*v*norm(v)*ro*S*c;
end

== matlab function forGenerate/control/ExtendedMellingerControl/Th, W/hyro propeller moment prediction/wp ==
  data: q_PB input; omegaP output; omegaB input; Th_dot input; W input
function omegaP  = fcn(q_PB, omegaB, Th_dot, W)

omegaP = zeros(4*3,1);
for i = 1:4
    
    q_pb = q_PB(:, i);
    q_bp = quatDual(q_pb);
    w = sign(W(i))*sqrt(abs(W(i)));
    omegaP(3*i-2:3*i, 1) = quatRotate(q_bp, omegaB) + [Th_dot(i); 0; w];
    w1 = [0;0;w];
    th1 = [Th_dot(i); 0; 0];
    Ob1 = quatRotate(q_bp, omegaB);
end
